simulink model "untitled"  (R2021a)
settings: Solver=VariableStepAuto  StartTime=0.0  StopTime=10.0  RelTol=1e-3
settings Model: Creator=oscar  LastModifiedBy=oscar

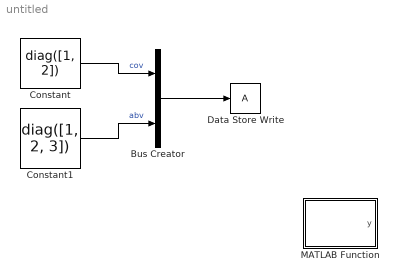
== system untitled ==
  Bus Creator : BusCreator  Inputs=2
  Constant : Constant  Value=diag([1, 2])
  Constant1 : Constant  Value=diag([1, 2, 3])
  Data Store Write : DataStoreWrite  IndexOptions=Index vector (dialog)  Indices=1  OutputSizes=1
  MATLAB Function : MATLAB Function  TreatAsAtomicUnit=on
  wires:
  Constant/1 -> Bus Creator/1  "cov"
  Constant1/1 -> Bus Creator/2  "abv"
  Bus Creator/1 -> Data Store Write/1

== matlab function untitled/MATLAB Function ==
  data: y output
function y = fcn()

global A;

A.cov = A.cov*2;
y = A.cov;
